simulink model "Virtual_Veh_Sim_EV3M_DLC"  (R2020a)
settings: configuration reference "Config_VarStep_Lat" (kept outside this file)
model workspace (MAT data in the model file):
  A = 159.22
  AccPwrbp = [0 0]
  AccSpdbp = [300 750]
  Aeff = 0.0314159265359
  Af = 2.46
  AfrStoich = 14.6
  AxlIxx = 62.3745166667
  AxlM = 160
  B = 1.01
  BattCapInit = 3.18
  BattCapInit_EV = 4.24
  BattChargeMax = 5.3
  BattChrgPwrMax = -60000
  BattChrgPwrMax_EV = -350000
  BattCurrMax = 300
  BattCurrMax_EV = 900
  BattDischrgPwrMax = 85000
  BattDischrgPwrMax_EV = 497000
  BattTempBp = [243.1 253.1 263.1 273.1 283.1 298.1 313.1]
  Battery : object (value not decoded)
  BrkPrsMax = 8273709
  Bx = 10
  C = 0.3618
  CapLUTBp = [0 0.01 0.02 0.03 0.04 0.05 0.06 0.07 0.08 0.09 0.1 0.11 ... (101 elements, 1x101)]
  CapSOCBp = [0 0.2 0.4 0.6 0.8 1]
  CatLightOffTime = 0
  Cd = 0.25
  ChrgLmt_bpt = [1 1 1 1 1 1 1 0.9 0.7 0.5 0]
  Cl = 0.1
  Cpm = 0.1
  Cps = 2
  CrankSpeed = 150
  Cx = 1.65
  Cz = 5565.2246438
  CzWhlAxl = 11490.971257
  DCT_Param : object (value not decoded)
  DischrgLmt_bpt = [0 0.5 0.7 0.9 1 1 1 1 1 1 1]
  Dn_Shft_Spd = [3 3 10 10 7 7 17 17 11 11 26 26 ... (20 elements, 4x5)]
  Downshift_Speeds = [9.5625 12.9375 16.3125 19.6875 23.0625 26.4375 29.8125 33.1875 36.5625 39.9375 43.3125 46.6875 ... (28 elements, 4x7)]
  Dx = 1
  ECMS_Ki = 0.1
  ECMS_Kp = 3
  ECMS_method = 1
  ECMS_s = 3.4
  Em = [2.8 3.228 3.284 3.361 3.408 3.427 3.472 3.477 3.493 3.504 3.516 3.528 ... (101 elements, 1x101)]
  EngStopStartEnable = 1
  EngStopTime : Simulink.Parameter (value not decoded)
  EngTrqCmd_0 = [0 5.91462851599 6.30130128159 6.63745773103 6.93103920513 7.1887141028 7.41614736865 7.6182009157 7.79908238179 7.96245469721 8.11151569725 8.24905488129 ... (21 elements, 1x21)]
  Ex = 0.01
  F0z = [2886 2907]
  F0zWhlAxl = 2907
  FZMAX = 6570
  FZMIN = 0
  Fc = 500
  FsbF = [-700000 -7000 -700 0 700 7000 700000]
  FsbR = [-700000 -7000 -700 0 700 7000 700000]
  FskF = [-8928.57142857 -178.571428571 0 357.142857143 535.714285714 9285.71428571]
  FskR = [-5357.14285714 -107.142857143 0 214.285714286 321.428571429 5571.42857143]
  G = [-1 0 1 2 3 4 5 6]
  G_o = 1
  Gear_Dn_bpt = [2 3 4 5 6]
  Gear_Up_bpt = [1 2 3 4 5]
  HEVEngTrq_min = 16.186104388
  Hmax = 0.25
  Iyy = 3000
  Iyy_Whl = 0.8
  J = 0.01
  J1 = 0.01
  J2 = 0.01
  Jd = 0.025
  Ji = 0.1
  Jin = 0.05
  Jin_Cltch = 0.2
  Jin_Cltch2 = 0.01
  Jout = [0.01 0.009 0.01 0.01 0.01 0.01 0.01 0.01]
  Jout_Cltch = 0.01
  Jout_Cltch2 = 0.05
  Jt = 0.1
  Jw1 = 0.01
  Jw2 = 0.01
  K_c = 10000
  Kpt = 12798
  Kz = 52451.0065793
  KzWhlAxl = 138031.612078
  LHV = 43000000
  Lhv = 42940000
  Lrel = 0.15
  Mass = 1623
  MaxTorque = [10.8721902117 76.2227873944 95.7133163788 115.203846226 134.694376076 154.184905918 173.675435766 181.839920951 181.509869828 181.17981871 180.849767971 180.519716854 ... (21 elements, 21x1)]
  N = [3.39 1 4.212 2.637 1.8 1.386 1 0.772]
  NCyl = 4
  NF = 2
  NR = 2
  N_P0 = 3
  N_P4 = 4.1
  N_idle = 750
  Ndiff = 3.32
  Ndiff_P4 = 4.1
  Ndiff_front = 5
  Ndiff_rear = 3.5
  Ndisk = 1
  Ndisks = 4
  Ngrid = 200
  Np = 2
  Np_EV = 35
  Np_FC = 1
  Ns = 72
  Ns_EV = 96
  Pabs = 101325
  Pdl_Pos_Dn_bpt = [0 0.6 0.9 1]
  Pdl_Pos_Up_bpt = [0 0.25 0.9 1]
  Pedal_Positions = [0.1 0.4 0.5 0.9]
  PenaltyFctr = 10000000
  Plimit = 60000
  Plimit_EV = 350000
  Press = 7000000
  Pstd = 101325
  RInt = [0.008846 0.006389 0.004364 0.002031 0.001443 0.0005603 0.001028 0.009319 0.006554 0.004101 0.002563 0.001825 ... (42 elements, 7x6)]
  Rair = 287
  Re = 0.327
  Reff = 0.11
  Reff_LSD = 0.2
  RegenBrkCutOff = [0 1]
  RegenBrkSpd_bpt = [2.2352 4.4704]
  Rm = 0.15
  SOCInit = 0.5
  SOCTrgt = 60
  SOC_bpt = [0 0.1 0.2 0.3 0.4 0.5 0.6 0.7 0.8 0.9 1]
  SOCmax = 80
  SOCmin = 40
  SUS : object (value not decoded)
  Sg = 0.743
  Sinj = 6.45161290323
  T = 273
  TCopy = 300
  T_eff_bp = [0 20 40 60 80 100 120 140 160 180 200]
  T_eff_bp_EV_front = [0 30 60 90 120 150 180 210 240 270 300]
  T_eff_bp_EV_rear = [0 20 40 60 80 100 120 140 160 180 200]
  T_eff_bp_P0 = [0 5.78745247607 6.36619772368 7.07355302631 7.95774715459 9.09456817668 10.6103295395 12.7323954474 15.9154943092 21.2206590789 66.6666666667]
  T_init = 298.15
  T_t = [200 200 200 200 190.9859317 143.2394488 114.591559 95.49296586 81.85111359 71.61972439 63.66197724 57.29577951 ... (14 elements, 1x14)]
  T_t_EV_front = [300 300 300 300 286.47889755 214.8591732 171.8873385 143.23944879 122.776670385 107.429586585 95.49296586 85.943669265 ... (14 elements, 1x14)]
  T_t_EV_rear = [200 200 200 200 190.9859317 143.2394488 114.591559 95.49296586 81.85111359 71.61972439 63.66197724 57.29577951 ... (14 elements, 1x14)]
  T_t_P0 = [66.6666666667 66.6666666667 66.6666666667 66.6666666667 21.2206590789 15.9154943092 12.7323954474 10.6103295395 9.09456817668 7.95774715459 7.07355302631 6.36619772368 ... (14 elements, 1x14)]
  Tc_Batt = 0.001
  Tc_DC = 0.001
  Tc_Mot = 0.02
  Temp_bpts = [313 358]
  TimeCnstECP = 0.125
  TimeCnstEGR = 0.125
  TimeCnstETC = 0.085
  TimeCnstICP = 0.125
  TimeCnstIVL = 0.125
  TimeCnstMFA = 0.125
  TimeCnstSWVA = 0.125
  TimeCnstVCR = 0.125
  TimeCnstVGT = 0.15
  TimeCnstVIRL = 0.125
  TimeCnstWGA = 0.15
  TimeStep = 0.0001
  TracPenaltyFctr = 50
  Trans : object (value not decoded)
  Trq_bpts = [25 50 75 100 150 200 250]
  Ts : Simulink.Parameter (value not decoded)
  Tstd = 293.15
  UNLOADED_RADIUS = 0.336
  Up_Shft_Spd = [5 5 12 12 9 9 19 19 13 13 28 28 ... (20 elements, 4x5)]
  Upshift_Speeds = [12.9375 16.3125 19.6875 33 26.4375 29.8125 33.1875 52.5 39.9375 43.3125 46.6875 77.25 ... (28 elements, 4x7)]
  VEH : object (value not decoded)
  VXLOW = 2
  Vd = 0.0015
  Vinit = 650
  WH : Mass (value not decoded)
  a = 3
  aMy = 0.01
  a_CG = 1.09
  afr_stoich = 14.6
  alphaMy = 0
  b : Simulink.Parameter (value not decoded)
  b1 = 100
  b1_g = 0.001
  b2 = 100
  b2_g = 0.001
  bMy = 0
  b_CG = 1.7
  b_J = 0.001
  bd = 0.001
  behavior = 0.2
  betaMy = 1
  bi = 0.001
  bin = 0.003
  bin_Cltch = 0.003
  bout = [0.003 0.003 0.003 0.003 0.003 0.003 0.003 0.003]
  bout_Cltch = 0.003
  br = 0.001
  bt = 0.001
  bw1 = 0.001
  bw2 = 0.001
  cMy = 0
  controller_type = 2
  defaultSpacing = 15
  disk_abore = 0.05
  domega_o = 0
  dt3D = 0.05
  dw = [0 10 20 40 60 80 100]
  dzdotsF = [-10 -1 -0.1 0 0.1 1 10]
  dzdotsR = [-10 -1 -0.1 0 0.1 1 10]
  dzsF = [-0.005 -0.0001 0 0.2 0.2001 0.2051]
  dzsR = [-0.005 -0.0001 0 0.2 0.2001 0.2051]
  eff = 98
  efficiency_table = [52 52 52 52 52 52 52 52 52 62 66 70 ... (154 elements, 14x11)]
  efficiency_table_EV = [85 85 85 85 85 85 85 85 85 85 85 85 ... (154 elements, 14x11)]
  efficiency_table_P0 = [52 52 52 52 52 52 52 52 52 62 66 70 ... (154 elements, 14x11)]
  egotf : object (value not decoded)
  elec_Pipe : object (value not decoded)
  elec_Radiator : object (value not decoded)
  eta = [0.95 0.95 0.95 0.95 0.95 0.95 0.95 0.95]
  eta_tbl = [0.7 0.8 0.9 0.9 0.9 0.9 0.9 0.7 0.8 0.9 0.9 0.9 ... (1232 elements, 7x11x8x2)]
  f_air = [0 0 0 0 0 0 0 0 0 0 0 0 ... (441 elements, 21x21)]
  f_co = [0 0 0 0 0 0 0 0 0 0 0 0 ... (441 elements, 21x21)]
  f_co2 = [0 0 0 0 0 0 0 0 0 0 0 0 ... (441 elements, 21x21)]
  f_cp_ld_bpt = [0 0.2 0.275 0.35 0.425 0.5 0.575 0.65 0.725 0.8 0.875 0.95 ... (16 elements, 1x16)]
  f_cp_n_bpt = [750 1053.57142857 1357.14285714 1660.71428571 1964.28571429 2267.85714286 2571.42857143 2875 3178.57142857 3482.14285714 3785.71428571 4089.28571429 ... (15 elements, 1x15)]
  f_del_sa_bpt = [0 0.75 1.5 2.25 3 3.75 4.5 5.25 6 6.75 7.5 8.25 ... (65 elements, 1x65)]
  f_ecp = [0 0 7.19012817097 15.3709456879 19.1470470057 19.0854874367 13.5819971805 0 0 0 0 0 ... (240 elements, 16x15)]
  f_eff = [499.877436556 432.508206156 399.540781628 370.894662993 347.954880181 331.11554878 319.468905906 311.408898718 305.523567029 300.961538912 297.204959405 293.79866205 ... (441 elements, 21x21)]
  f_egr_areapct_cmd = [0 3.448 6.897 10.34 13.79 17.24 20.69 24.14 27.59 31.03 34.48 37.93 ... (600 elements, 30x20)]
  f_egr_areapct_nrmlzdflow_bpt = [0 0.03448 0.06897 0.1034 0.1379 0.1724 0.2069 0.2414 0.2759 0.3103 0.3448 0.3793 ... (30 elements, 1x30)]
  f_egr_areapct_pr_bpt = [0.5 0.5263 0.5526 0.5789 0.6053 0.6316 0.6579 0.6842 0.7105 0.7368 0.7632 0.7895 ... (20 elements, 20x1)]
  f_egr_max_stdflow = [74.87 74.87 74.74 74.39 73.81 72.98 71.91 70.58 68.97 67.06 64.84 62.25 ... (20 elements, 1x20)]
  f_egr_stdflow = [0 3.743 7.487 11.23 14.97 18.72 22.46 26.2 29.95 33.69 37.43 41.18 ... (420 elements, 21x20)]
  f_egr_stdflow_egrap_bpt = [0 5 10 15 20 25 30 35 40 45 50 55 ... (21 elements, 21x1)]
  f_egr_stdflow_pr_bpt = [0.5 0.5263 0.5526 0.5789 0.6053 0.6316 0.6579 0.6842 0.7105 0.7368 0.7632 0.7895 ... (20 elements, 20x1)]
  f_egrpct_cmd = [0 0 0 0 0 0 0 0 0 0 0 0 ... (240 elements, 16x15)]
  f_egrpct_ld_bpt = [0 0.2 0.275 0.35 0.425 0.5 0.575 0.65 0.725 0.8 0.875 0.95 ... (16 elements, 1x16)]
  f_egrpct_n_bpt = [750 1054 1357 1661 1964 2268 2571 2875 3179 3482 3786 4089 ... (15 elements, 1x15)]
  f_fric_temp_bpt = [275 277 279 281 283 285 287 289 291 293 295 297 ... (46 elements, 1x46)]
  f_fric_temp_mod = [3.986 2.616 2.132 1.946 1.839 1.747 1.672 1.608 1.551 1.499 1.462 1.415 ... (46 elements, 1x46)]
  f_fuel = [0 0 0 0 0 0 0 0 0 0 0 0 ... (441 elements, 21x21)]
  f_hc = [0 0 0 0 0 0 0 0 0 0 0 0 ... (441 elements, 21x21)]
  f_icp = [0 0 1 1.09273642197 2.29409401139 3.54274371837 0.947749647567 0 0 0 0 0 ... (240 elements, 16x15)]
  f_intksys_stdflow_bpt = [0 29.67 59.34 89.01 117.8 144.1 155.7 166 175.2 183.3 190.7 197 ... (20 elements, 1x20)]
  f_intksys_stdflow_pr = [1 0.9789 0.9579 0.9368 0.9158 0.8947 0.8737 0.8526 0.8316 0.8105 0.7895 0.7684 ... (20 elements, 1x20)]
  f_lamcmd = [1 1 1 1 1 1 1 1 1 1 1 1 ... (240 elements, 16x15)]
  f_lamcmd_ld_bpt = [0 0.2 0.275 0.35 0.425 0.5 0.575 0.65 0.725 0.8 0.875 0.95 ... (16 elements, 1x16)]
  f_lamcmd_n_bpt = [750 1053.57142857 1357.14285714 1660.71428571 1964.28571429 2267.85714286 2571.42857143 2875 3178.57142857 3482.14285714 3785.71428571 4089.28571429 ... (15 elements, 1x15)]
  f_lcmd = [0 0.323404450126 0.402272754123 0.472190900601 0.545782048677 0.619112163094 0.619299299836 0.619299299836 0.619299299836 0.619299299836 0.619299299836 0.619299299836 ... (315 elements, 21x15)]
  f_lcmd_n_bpt = [750 1053.57142857 1357.14285714 1660.71428571 1964.28571429 2267.85714286 2571.42857143 2875 3178.57142857 3482.14285714 3785.71428571 4089.28571429 ... (15 elements, 1x15)]
  f_lcmd_tq_bpt = [0 15 25.2631578947 35.5263157895 45.7894736842 56.0526315789 66.3157894737 76.5789473684 86.8421052632 97.1052631579 107.368421053 117.631578947 ... (21 elements, 1x21)]
  f_m_lam = [0.94128 0.95565 0.97001 0.98437 0.99008 1.0004 0.97527 0.9549 0.92612 0.89735]
  f_m_lam_bpt = [0.65 0.7 0.75 0.8 0.85 0.9 0.95 1 1.05 1.1]
  f_m_sa = [1.0019 0.9988 0.9953 0.99173 0.98811 0.98441 0.98065 0.97682 0.97293 0.96897 0.96493 0.96083 ... (65 elements, 1x65)]
  f_mdot_air_corr = [1.02156051768 1.00597426471 0.989411677851 1.0033499089 0.984591437857 0.988509040623 1.0326198627 1.02765527362 1.0134784519 0.998280021213 0.981755128787 0.967218261288 ... (400 elements, 20x20)]
  f_mdot_air_corr_ld_bpt = [0.223381333333 0.285105122807 0.346828912281 0.408552701754 0.470276491228 0.532000280702 0.593724070175 0.655447859649 0.717171649123 0.778895438596 0.84061922807 0.902343017544 ... (20 elements, 1x20)]
  f_mdot_air_n_bpt = [750 973.6842 1197.3684 1421.0526 1644.7368 1868.4211 2092.1053 2315.7895 2539.4737 2763.1579 2986.8421 3210.5263 ... (20 elements, 1x20)]
  f_mdot_intk = [0 0 0 0 0 0 0 0 0 0 0 0 ... (400 elements, 20x20)]
  f_mdot_intk_ecp_bpt = [0 2.6316 5.2632 7.8947 10.5263 13.1579 15.7895 18.4211 21.0526 23.6842 26.3158 28.9474 ... (20 elements, 1x20)]
  f_mdot_trpd_bpt = [0 5.7895 11.5789 17.3684 23.1579 28.9474 34.7368 40.5263 46.3158 52.1053 57.8947 63.6842 ... (20 elements, 1x20)]
  f_nox = [0 0 0 0 0 0 0 0 0 0 0 0 ... (441 elements, 21x21)]
  f_nv = [0.64175366561 0.641419295169 0.640125365558 0.638690556197 0.644169906538 0.669178791311 0.731659452876 0.750078238889 0.750078238889 0.750078238889 0.750078238889 0.750078238889 ... (225 elements, 15x15)]
  f_nv_n_bpt = [750 1053.57142857 1357.14285714 1660.71428571 1964.28571429 2267.85714286 2571.42857143 2875 3178.57142857 3482.14285714 3785.71428571 4089.28571429 ... (15 elements, 1x15)]
  f_nv_prs_bpt = [31 40.6428571429 50.2857142857 59.9285714286 69.5714285714 79.2142857143 88.8571428571 98.5 108.142857143 117.785714286 127.428571429 137.071428571 ... (15 elements, 1x15)]
  f_pm = [0 0 0 0 0 0 0 0 0 0 0 0 ... (441 elements, 21x21)]
  f_sa = [9.05 9.05 16.4373253582 15.3405265461 13.6074880273 9.83352189562 3.89388784387 0 0 0 0 0 ... (240 elements, 16x15)]
  f_sa_ld_bpt = [0 0.2 0.275 0.35 0.425 0.5 0.575 0.65 0.725 0.8 0.875 0.95 ... (16 elements, 1x16)]
  f_sa_n_bpt = [750 1053.57142857 1357.14285714 1660.71428571 1964.28571429 2267.85714286 2571.42857143 2875 3178.57142857 3482.14285714 3785.71428571 4089.28571429 ... (15 elements, 1x15)]
  f_sa_opt = [35.3085 21.0105 10.3714 8.5076 7.1426 7.5656 -5.7766 -16.7061 -16.8345 -19.3546 -20.6085 -22.0872 ... (225 elements, 15x15)]
  f_startup_ect_bpt = [-40 0 20 50]
  f_startup_lambda_delta = [0.5 0.3 0.2 0]
  f_startup_lambda_delta_timecnst = [90 40 12 0]
  f_susp_axl_bp = [1 2]
  f_susp_dz_bp = [-0.325022776267 -0.315022776267 -0.305022776267 -0.205022776267 -0.105022776267 -0.00502277626717 0.0949772237328 0.194977223733 0.204977223733 0.214977223733]
  f_susp_dzdot_bp = [-3 -0.3 -0.2 -0.1 0 0.1 0.2 0.3 3]
  f_susp_fmz = [-144070.391448 -93629.24037 -75929.1118915 -20630.5828179 -15385.48216 -10140.3815021 -4895.28084414 349.819813785 -31916.3973792 18437.6709544 -83996.1993354 -33555.0482577 ... (43920 elements, 10x9x61x2x4)]
  f_susp_geom = [0 0 0 0 0 0 0 0 0 0 0 0 ... (3660 elements, 10x61x2x3)]
  f_susp_strgdelta_bp = [-0.523598775598 -0.506145483078 -0.488692190558 -0.471238898038 -0.453785605519 -0.436332312999 -0.418879020479 -0.401425727959 -0.383972435439 -0.366519142919 -0.349065850399 -0.331612557879 ... (61 elements, 1x61)]
  f_t_exh = [739.936218766 750.584766028 772.770773797 791.235245621 803.106549716 885.862998064 920.498479307 920.498479307 920.498479307 920.498479307 920.498479307 920.498479307 ... (225 elements, 15x15)]
  f_t_exh_l_bpt = [0.2 0.275 0.35 0.425 0.5 0.575 0.65 0.725 0.8 0.875 0.95 1.025 ... (15 elements, 1x15)]
  f_t_exh_n_bpt = [750 1053.57142857 1357.14285714 1660.71428571 1964.28571429 2267.85714286 2571.42857143 2875 3178.57142857 3482.14285714 3785.71428571 4089.28571429 ... (15 elements, 1x15)]
  f_tap = [0 0.9375 0.9375 0.982121188204 1.22093639741 1.5421156717 1.98870690459 2.59666257968 2.6875 2.6875 2.6875 2.6875 ... (315 elements, 21x15)]
  f_tap_ld_bpt = [0 0.2 0.268421052632 0.336842105263 0.405263157895 0.473684210526 0.542105263158 0.610526315789 0.678947368421 0.747368421053 0.815789473684 0.884210526316 ... (21 elements, 1x21)]
  f_tap_n_bpt = [750 1053.57142857 1357.14285714 1660.71428571 1964.28571429 2267.85714286 2571.42857143 2875 3178.57142857 3482.14285714 3785.71428571 4089.28571429 ... (15 elements, 1x15)]
  f_tbrake = [0 10.8721902117 10.8721902117 10.8721902117 10.8721902117 10.8721902117 10.8721902117 10.8721902117 10.8721902117 10.8721902117 10.8721902117 10.8721902117 ... (441 elements, 21x21)]
  f_tbrake_n_bpt = [0 750 973.684210526 1197.36842105 1421.05263158 1644.73684211 1868.42105263 2092.10526316 2315.78947368 2539.47368421 2763.15789474 2986.84210526 ... (21 elements, 1x21)]
  f_tbrake_t_bpt = [0 16.186104388 24.9146526824 33.6432009767 42.3717492711 51.1002975655 59.8288458599 68.5573941543 77.2859424487 86.0144907431 94.7430390375 103.471587332 ... (21 elements, 21x1)]
  f_texh = [630.359790352 638.212816583 644.85156876 656.410931683 676.180276582 706.880985433 749.880156186 804.757804763 869.00210738 938.264388175 1007.38061415 1071.70023123 ... (441 elements, 21x21)]
  f_tm_corr = [0.839360054391 0.833393271885 0.82629554201 0.818442814437 0.811524387436 0.809164184856 0.814606352881 0.826887956871 0.842304598924 0.856886829014 0.869487025783 0.880530414174 ... (400 elements, 20x20)]
  f_tm_corr_n_bpt = [750 973.6842 1197.3684 1421.0526 1644.7368 1868.4211 2092.1053 2315.7895 2539.4737 2763.1579 2986.8421 3210.5263 ... (20 elements, 1x20)]
  f_tm_corr_nd_bpt = [0.3 0.38947 0.47895 0.56842 0.65789 0.74737 0.83684 0.92632 1.0158 1.1053 1.1947 1.2842 ... (20 elements, 1x20)]
  f_tpp = [0 100]
  f_tpp_tap_bpt = [0 100]
  f_tq_fric = [4.16 4.42 4.69 4.88 4.94 4.93 4.85 4.74 4.63 4.52 4.42 4.34 ... (225 elements, 15x15)]
  f_tq_inr = [25.8508 37.8267 50.6081 62.6825 74.6026 88.9064 81.9508 76.6399 82.9886 85.0042 88.9209 92.7645 ... (225 elements, 15x15)]
  f_tq_inr_l_bpt = [0.2 0.28571 0.37143 0.45714 0.54286 0.62857 0.71429 0.8 0.88571 0.97143 1.0571 1.1429 ... (15 elements, 1x15)]
  f_tq_inr_n_bpt = [750 1053.5714 1357.1429 1660.7143 1964.2857 2267.8571 2571.4286 2875 3178.5714 3482.1429 3785.7143 4089.2857 ... (15 elements, 1x15)]
  f_tq_nl = [0 15.0012133443 26.4298333923 37.8556656512 49.2846782956 60.7113978793 72.3451969202 77.459652163 78.5324534074 78.5324534074 78.5324534074 78.5324534074 ... (256 elements, 16x16)]
  f_tq_nl_l_bpt = [0 0.2 0.275 0.35 0.425 0.5 0.575 0.65 0.725 0.8 0.875 0.95 ... (16 elements, 1x16)]
  f_tq_nl_n_bpt = [0 750 1053.57142857 1357.14285714 1660.71428571 1964.28571429 2267.85714286 2571.42857143 2875 3178.57142857 3482.14285714 3785.71428571 ... (16 elements, 1x16)]
  f_tq_pump = [7.24 5.67 3.94 2.59 1.8 1 1 1 1 1 1 1 ... (225 elements, 15x15)]
  f_twc_eff_co = [0.17 0.25 0.45 0.99 0.99 0.99 0.99]
  ... (+78 more variables)
symbols that are objects in the model workspace (value not decoded): VEH
undefined symbols (not defined in the file or in its folder): Disabled, DLCXref, DLCYref, Right, sigbuilder_block, SRE
libraries: simulink x11, vehdynlibscenariocommon x5, simulink_extras x5, vrlib x2, sim3dlib x2, vehdynlibviscommon x2, autolibshared x1, vehdynlibdriver x1, sim3dautolib x1
(part 4 of 6)

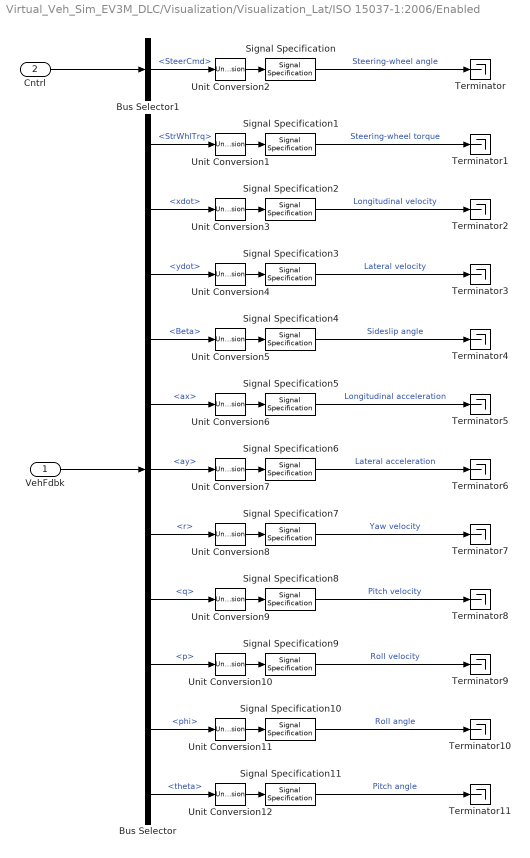
== system Virtual_Veh_Sim_EV3M_DLC/Visualization/Visualization_Lat/ISO 15037-1:2006/Enabled ==
  VehFdbk : Inport
  Cntrl : Inport  Port=2
  Bus Selector : BusSelector  OutputSignals=Steering.StrWhlTrq,Body.xdot,Body.ydot,Body.Beta,Body.ax,Body.ay,Body.r,Body.q,Body.p,Body.phi,Body.theta
  Bus Selector1 : BusSelector  OutputSignals=SteerCmd
  Signal Specification{,4,10..11} (4 alike) : SignalSpecification  Unit=deg
  Signal Specification1 : SignalSpecification  Unit=N*m
  Signal Specification2 : SignalSpecification  Unit=km/h
  Signal Specification3 : SignalSpecification  Unit=m/s
  Signal Specification5 : SignalSpecification  Unit=m/s^2
  Signal Specification6 : SignalSpecification  Unit=m/s^2
  Signal Specification7 : SignalSpecification  Unit=deg/s
  Signal Specification8 : SignalSpecification  Unit=deg/s
  Signal Specification9 : SignalSpecification  Unit=deg/s
  Terminator{,1..11} (12 alike) : Terminator
  Unit Conversion{1..12} (12 alike) : UnitConversion
  wires:
  Bus Selector/11 -> Unit Conversion12/1  "<theta>"
  Signal Specification11/1 -> Terminator11/1  "Pitch angle"
  Unit Conversion12/1 -> Signal Specification11/1
  Bus Selector/10 -> Unit Conversion11/1  "<phi>"
  Unit Conversion11/1 -> Signal Specification10/1
  Signal Specification10/1 -> Terminator10/1  "Roll angle"
  Bus Selector/9 -> Unit Conversion10/1  "<p>"
  Signal Specification9/1 -> Terminator9/1  "Roll velocity"
  Unit Conversion10/1 -> Signal Specification9/1
  Bus Selector/8 -> Unit Conversion9/1  "<q>"
  Unit Conversion9/1 -> Signal Specification8/1
  Signal Specification8/1 -> Terminator8/1  "Pitch velocity"
  Bus Selector/7 -> Unit Conversion8/1  "<r>"
  Signal Specification7/1 -> Terminator7/1  "Yaw velocity"
  Unit Conversion8/1 -> Signal Specification7/1
  Bus Selector/6 -> Unit Conversion7/1  "<ay>"
  Unit Conversion7/1 -> Signal Specification6/1
  Signal Specification6/1 -> Terminator6/1  "Lateral acceleration"
  Bus Selector/5 -> Unit Conversion6/1  "<ax>"
  Signal Specification5/1 -> Terminator5/1  "Longitudinal acceleration"
  Unit Conversion6/1 -> Signal Specification5/1
  Bus Selector/4 -> Unit Conversion5/1  "<Beta>"
  Unit Conversion5/1 -> Signal Specification4/1
  Signal Specification4/1 -> Terminator4/1  "Sideslip angle"
  Bus Selector/3 -> Unit Conversion4/1  "<ydot>"
  Signal Specification3/1 -> Terminator3/1  "Lateral velocity"
  Unit Conversion4/1 -> Signal Specification3/1
  Bus Selector/2 -> Unit Conversion3/1  "<xdot>"
  Unit Conversion3/1 -> Signal Specification2/1
  Signal Specification2/1 -> Terminator2/1  "Longitudinal velocity"
  Signal Specification1/1 -> Terminator1/1  "Steering-wheel torque"
  Unit Conversion1/1 -> Signal Specification1/1
  Bus Selector/1 -> Unit Conversion1/1  "<StrWhlTrq>"
  Signal Specification/1 -> Terminator/1  "Steering-wheel angle"
  Unit Conversion2/1 -> Signal Specification/1
  Bus Selector1/1 -> Unit Conversion2/1  "<SteerCmd>"
  Cntrl/1 -> Bus Selector1/1
  VehFdbk/1 -> Bus Selector/1

== system Virtual_Veh_Sim_EV3M_DLC/Visualization/Visualization_Lat/Scope Type/DLC ==
  VehFdbk : Inport
  Vis : Inport  Port=2
  Bus Creator : BusCreator  Inputs=3
  Bus Selector3 : BusSelector  OutputSignals=Veh.Body.Y,Veh.Body.X,Veh.Body.Z
  Bus Selector4 : BusSelector  OutputSignals=UB,LB,LtrlRef
  Lane Change : Scope  Commented=on
  Mux1 : Mux  Commented=on
  Signal Copy : SignalConversion  OverrideOpt=off
  Signal Copy1 : SignalConversion  OverrideOpt=off
  Signal Copy2 : SignalConversion  OverrideOpt=off
  Ref : Outport  VectorParamsAs1DForOutWhenUnconnected=off
  wires:
  Bus Selector4/1 -> Mux1/1  "<UB>"
  Bus Selector3/1 -> Mux1/4  "<Y>"
  VehFdbk/1 -> Bus Selector3/1
  Mux1/1 -> Lane Change/1
  Vis/1 -> Bus Selector4/1
  Bus Selector4/3 -> Signal Copy/1, Mux1/3  "<LtrlRef>"
  Bus Selector4/2 -> Mux1/2  "<LB>"
  Bus Selector3/2 -> Signal Copy1/1  "<X>"
  Bus Creator/1 -> Ref/1
  Bus Selector3/3 -> Signal Copy2/1  "<Z>"
  Signal Copy/1 -> Bus Creator/2  "YRef"
  Signal Copy1/1 -> Bus Creator/1  "XRef"
  Signal Copy2/1 -> Bus Creator/3  "ZRef"

== system Virtual_Veh_Sim_EV3M_DLC/Visualization/Visualization_Lat/Scope Type/None ==
  VehFdbk : Inport
  Vis : Inport  Port=2
  Cntrl : Inport  Port=3
  Bus Selector1 : BusSelector  OutputSignals=SteerCmd
  Bus Selector9 : BusSelector  OutputSignals=Veh.Body.r
  Signal Specification3 : SignalSpecification  Unit=deg/s
  Unit Conversion4 : UnitConversion
  Yaw Rate and Steer : Scope  NumInputPorts=2
  Ref : Outport  VectorParamsAs1DForOutWhenUnconnected=off
  wires:
  Bus Selector9/1 -> Unit Conversion4/1  "<r>"
  Signal Specification3/1 -> Yaw Rate and Steer/1
  Unit Conversion4/1 -> Signal Specification3/1
  VehFdbk/1 -> Bus Selector9/1  "VehFdbk"
  Bus Selector1/1 -> Yaw Rate and Steer/2  "<SteerCmd>"
  Vis/1 -> Ref/1
  Cntrl/1 -> Bus Selector1/1

== system Virtual_Veh_Sim_EV3M_DLC/Visualization/Visualization_Lat/Scope Type/XYZ ==
  VehFdbk : Inport
  Vis : Inport  Port=2
  Terminator : Terminator
  Ref : Outport  VectorParamsAs1DForOutWhenUnconnected=off
  wires:
  Vis/1 -> Ref/1
  VehFdbk/1 -> Terminator/1

== system Virtual_Veh_Sim_EV3M_DLC/Visualization/Visualization_Lat/Vehicle XY Plotter/XY View ==
  VehFdbk : Inport
  Bus Selector1 : BusSelector  OutputSignals=Veh.Body.phi,Veh.Body.theta,Veh.Body.psi  OutputAsBus=on
  Bus Selector5 : BusSelector  OutputSignals=Veh.Wheels.WhlAng  OutputAsBus=on
  Bus Selector6 : BusSelector  OutputSignals=Veh.Body.GeomX,Veh.Body.GeomY,Veh.Body.GeomZ  OutputAsBus=on
  Bus Selector7 : BusSelector  OutputSignals=Veh.Body.GeomXdot,Veh.Body.GeomYdot,Veh.Body.GeomZdot  OutputAsBus=on
  Bus to Vector : BusToVector
  Bus to Vector1 : BusToVector
  Bus to Vector2 : BusToVector
  Vehicle XY Plotter : Subsystem  mask(Vehicle XY Plotter){a=VEH.FrontAxlePositionfromCG, b=VEH.RearAxlePositionfromCG, w=VEH.TrackWidth, figBorder=10, bufferSize=1024, extRef=off, pltDT=.1}
      mask prompts: a "Distance to front axle from CG, a [m]:"; b "Distance to rear axle from CG, b [m]:"; w "Track width, w [m]:"; figBorder "Distance to figure borders, figBorder [m]:"; bufferSize "Path buffer sampe size, bufferSize []:"; extRef "Plot path reference, extRef"; pltDT "Plot update rate, pltDT [s]:"
      mask help:
      | This block will display a MATLAB figure which indicates the vehicle path, current position and heading velocity.
      | An optional path reference is also provided.
      mask init:
      | if autoblkschecksimstopped(gcb)
      |     PortName = 'RefXYZ';
      |     InportOption  = {'built-in/Ground', [PortName, ' Ground'];...
      |         'built-in/Inport',PortName };
      |     if ~strcmp(get_param(gcb,'extRef'),'on')
      |         NewBlkHdl = autoblksreplaceblock(gcb, InportOption, 1);
      |         set_param(NewBlkHdl, 'ShowName', 'off');
      |     else
      |         autoblksreplaceblock(gcb, InportOption, 2);
      |     end
      | end
      mask TypeOptions a: Vehicle XY Plotter/a
      mask TypeOptions b: Vehicle XY Plotter/b
      mask TypeOptions w: Vehicle XY Plotter/w
      mask TypeOptions figBorder: Vehicle XY Plotter/figBorder
      mask TypeOptions bufferSize: Vehicle XY Plotter/bufferSize
  wires:
  Bus to Vector2/1 -> Vehicle XY Plotter/2(InertAng)
  Bus to Vector/1 -> Vehicle XY Plotter/1(InertXYZ)
  Bus Selector5/1 -> Vehicle XY Plotter/4(delta)
  Bus Selector1/1 -> Bus to Vector2/1
  Bus Selector6/1 -> Bus to Vector/1
  Bus Selector7/1 -> Bus to Vector1/1
  VehFdbk/1 -> Bus Selector6/1, Bus Selector1/1, Bus Selector7/1, Bus Selector5/1
  Bus to Vector1/1 -> Vehicle XY Plotter/3(InertXdotYdotZdot)

== system Virtual_Veh_Sim_EV3M_DLC/Visualization/Visualization_Lat/Vehicle XY Plotter/XY View Ref ==
  VehFdbk : Inport
  Ref : Inport  Port=2
  Bus Selector1 : BusSelector  OutputSignals=Veh.Body.phi,Veh.Body.theta,Veh.Body.psi  OutputAsBus=on
  Bus Selector5 : BusSelector  OutputSignals=Veh.Wheels.WhlAng  OutputAsBus=on
  Bus Selector6 : BusSelector  OutputSignals=Veh.Body.GeomX,Veh.Body.GeomY,Veh.Body.GeomZ  OutputAsBus=on
  Bus Selector7 : BusSelector  OutputSignals=Veh.Body.GeomXdot,Veh.Body.GeomYdot,Veh.Body.GeomZdot  OutputAsBus=on
  Bus Selector8 : BusSelector  OutputSignals=XRef,YRef,ZRef  OutputAsBus=on
  Bus to Vector{,1..3} (4 alike) : BusToVector
  Vehicle XY Plotter : Subsystem  mask(Vehicle XY Plotter){a=VEH.FrontAxlePositionfromCG, b=VEH.RearAxlePositionfromCG, w=VEH.TrackWidth, figBorder=10, bufferSize=1024, extRef=on, pltDT=.1}
      mask prompts: a "Distance to front axle from CG, a [m]:"; b "Distance to rear axle from CG, b [m]:"; w "Track width, w [m]:"; figBorder "Distance to figure borders, figBorder [m]:"; bufferSize "Path buffer sampe size, bufferSize []:"; extRef "Plot path reference, extRef"; pltDT "Plot update rate, pltDT [s]:"
      mask help:
      | This block will display a MATLAB figure which indicates the vehicle path, current position and heading velocity.
      | An optional path reference is also provided.
      mask init: same as Virtual_Veh_Sim_EV3M_DLC/Visualization/Visualization_Lat/Vehicle XY Plotter/XY View/Vehicle XY Plotter
      mask TypeOptions a: Vehicle XY Plotter/a
      mask TypeOptions b: Vehicle XY Plotter/b
      mask TypeOptions w: Vehicle XY Plotter/w
      mask TypeOptions figBorder: Vehicle XY Plotter/figBorder
      mask TypeOptions bufferSize: Vehicle XY Plotter/bufferSize
  wires:
  Bus Selector8/1 -> Bus to Vector3/1
  Bus to Vector1/1 -> Vehicle XY Plotter/3(InertXdotYdotZdot)
  VehFdbk/1 -> Bus Selector5/1, Bus Selector7/1, Bus Selector1/1, Bus Selector6/1
  Bus Selector7/1 -> Bus to Vector1/1
  Bus Selector6/1 -> Bus to Vector/1
  Bus Selector1/1 -> Bus to Vector2/1
  Bus Selector5/1 -> Vehicle XY Plotter/4(delta)
  Bus to Vector/1 -> Vehicle XY Plotter/1(InertXYZ)
  Bus to Vector2/1 -> Vehicle XY Plotter/2(InertAng)
  Ref/1 -> Bus Selector8/1
  Bus to Vector3/1 -> Vehicle XY Plotter/5(RefXYZ)

== system Virtual_Veh_Sim_EV3M_DLC/Driver/Lateral Ref + DRV/Driver Commands/Driver Commands/Longitudinal Driver ==
  note: Balance = 0
      | Charge = 1
      | Driving = 2
  VehRef : Inport
  VehFdbk : Inport  Port=2
  Bus Creator1 : BusCreator  Inputs=9
  Bus Selector : BusSelector  OutputSignals=Veh.Body.xdot
  Bus Selector1 : BusSelector  OutputSignals=SteerOvrCmd,LngRef
  Constant5 : Constant  Value=false
  Constant6 : Constant  Value=0  OutDataTypeStr=double
  Constant7 : Constant  OutDataTypeStr=double
  Data Type Conversion : DataTypeConversion  OutDataTypeStr=boolean
  Dead Zone : DeadZone  LowerValue=-.1  UpperValue=.1  SaturateOnIntegerOverflow=on
  Enumerated Constant : simulink/Sources/Enumerated Constant  OutDataTypeStr=Enum: SRE  Value=SRE.Driving  SampleTime=inf
  Ground : Ground
  Ignition Switch Profile1 : Subsystem  Tag=STV Subsys  LoadFcn=sigbuilder_block('load');  StartFcn=sigbuilder_block('start');  StopFcn=sigbuilder_block('stop');  ClipboardFcn=sigbuilder_block('clipboard');  mask(Sigbuilder block){tuvar=[0:10]}
      mask help: Simulink:masks:SigbuilderBlock_MD
      mask init:
      | if ~strcmp(get_param(bdroot(gcbh),'SimulationStatus'),'stopped') tuvar = sigbuilder_block('maskInit'); end
      settings: CopyFcn=sigbuilder_block('copy');  DeleteFcn=sigbuilder_block('delete');  ModelCloseFcn=sigbuilder_block('modelClose');  PreSaveFcn=sigbuilder_block('preSave');  PauseFcn=sigbuilder_block('pause');  ContinueFcn=sigbuilder_block('continue');  NameChangeFcn=sigbuilder_block('namechange');  OpenFcn=sigbuilder_block('open',[595.8 176.4 550.8 322.2 ]);  CloseFcn=sigbuilder_block('close');
      mask Display: plot(0, 0, 100, 100,[2, 2, 32, 32, 2], [68, 8, 8, 68, 68],[32, 2], [38, 38], [32, 19, 2],[53, 60, 44], [32, 17, 17, 2],[16, 16, 31, 31]);txt = getActiveGroup(gcbh);text(2, 100, txt,'verticalAlignment', 'top');
  Longitudinal Driver : autolibshared/Longitudinal Driver  extAccelOvr=off  extDecelOvr=off  extAccelHld=off  extDecelHld=off  extAccelZero=off  extDecelZero=off  cntrlType=Predictive  shftType=None  velUnits=m/s  gearOut=on  Kp=5  Ki=5  Kff=.1  Kg=0  VehVelVec=[0 100]  KffVec=[.1 .1]  KpVec=[10 10]  KiVec=[5 5]  KgVec=[0 0]  m=VEH.Mass  Kpt=20000*1.5  tau=.5  L=3  aR=200  bR=2.5  cR=.5  g=9.81  vnom=5  Kaw=1  tauerr=.1  tauPt=2  GearInit=0  tShift=.1  pdlVec=[0.1 0.4 0.5 0.9]  upShftTbl=[-1 12.9375 26.4375 39.9375 51.18749999999999 62.4375 72.84375 83.25;-1 16.3125 29.8125 43.3125 54.5624 65.8125 76.78125 87.75;-1 19.6875 33.1875 46.68749999999999 57.9375 69.1875 80.71875 92.25;-1 33 52.5 77.25 100.5 138.75 161.875 185]  dwnShftTbl=[1 9.5625 23.0625 36.5625 47.8125 59.0625 68.90625 78.75;1 12.9375 26.4375 39.9375 51.18749999999999 62.4375 72.84375 83.25;1 16.3125 29.8125 43.3125 54.562499 65.8125 76.78125 87.75;1 19.6875 33.1875 46.68749999999999 57.9375 69.1875 80.71875 92.25]  tClutch=.5  tRev=.5  tPark=120  aMode=2  UpGearVec="[0  1  2  3  4  5  6  7]"  DownGearVec="[1  2  3  4  5  6  7  8]"
      settings: SourceProductBaseCode=PW,MT,VE,VP
  Manual Switch : ManualSwitch
  Manual Switch1 : ManualSwitch
  Optional Stationary Charging : Subsystem  Commented=on
  Signal Specification3 : SignalSpecification  Unit=rad
  Subsystem1 : Subsystem
  Terminator3 : Terminator
  Unit Conversion : UnitConversion
  Driver : Outport  VectorParamsAs1DForOutWhenUnconnected=off
  wires:
  Dead Zone/1 -> Longitudinal Driver/2
  Bus Creator1/1 -> Driver/1
  Unit Conversion/1 -> Signal Specification3/1
  Longitudinal Driver/3 -> Bus Creator1/3  "Decel"
  Longitudinal Driver/1 -> Terminator3/1
  Bus Selector1/2 -> Longitudinal Driver/1  "<LngRef>"
  VehRef/1 -> Bus Selector1/1
  VehFdbk/1 -> Bus Selector/1
  Bus Selector/1 -> Dead Zone/1  "<xdot>"
  Longitudinal Driver/2 -> Bus Creator1/2  "Accel"
  Ground/1 -> Longitudinal Driver/3
  Longitudinal Driver/4 -> Bus Creator1/4  "Gear"
  Bus Selector1/1 -> Unit Conversion/1  "<SteerOvrCmd>"
  Data Type Conversion/1 -> Manual Switch/2
  Constant7/1 -> Manual Switch1/2
  Ignition Switch Profile1/1(IGSW) -> Data Type Conversion/1
  Constant5/1 -> Manual Switch/1
  Optional Stationary Charging/1(Charge) -> Bus Creator1/7  "Chrg"
  Constant6/1 -> Manual Switch1/1
  Manual Switch/1 -> Bus Creator1/6  "IgSw"
  Manual Switch1/1 -> Bus Creator1/5  "AccEnbl"
  Signal Specification3/1 -> Bus Creator1/1  "SteerCmd"
  Subsystem1/1(ShiftCmd) -> Bus Creator1/8
  Enumerated Constant/1 -> Bus Creator1/9  "BMS_StateRequest"

== system Virtual_Veh_Sim_EV3M_DLC/Driver/Lateral Ref + DRV/Driver Commands/Driver Commands/Open Loop - F310 Gamepad ==
  note: Balance = 0
      | Charge = 1
      | Driving = 2
  VehFdbk : Inport
  Bus Creator1 : BusCreator  Inputs=10
  Enumerated Constant : simulink/Sources/Enumerated Constant  OutDataTypeStr=Enum: SRE  Value=SRE.Driving  SampleTime=inf
  Ground{,1..3} (4 alike) : Ground
  Joystick Input : vrlib/Joystick Input  joyid=1  adjustports=on  forcefeed=off
  Subsystem : Subsystem
  Subsystem1 : Subsystem
  Terminator : Terminator
  To Workspace1 : ToWorkspace  Commented=on  VariableName=str_ref  SaveFormat=Timeseries  SampleTime=.01
  To Workspace2 : ToWorkspace  Commented=on  VariableName=acc_ref  SaveFormat=Timeseries  SampleTime=.01
  To Workspace3 : ToWorkspace  Commented=on  VariableName=brk_ref  SaveFormat=Timeseries  SampleTime=.01
  Driver : Outport  VectorParamsAs1DForOutWhenUnconnected=off
  wires:
  VehFdbk/1 -> Subsystem1/1(VehFdbk)
  Subsystem1/3(Brake) -> To Workspace3/1, Bus Creator1/7  "Decel"
  Subsystem1/2(Accel) -> To Workspace2/1, Bus Creator1/6  "Accel"
  Subsystem1/4(Clutch) -> Bus Creator1/8
  Subsystem1/1(Steer) -> To Workspace1/1, Bus Creator1/5  "SteerCmd"
  Joystick Input/2 -> Subsystem/1(In1)
  Ground1/1 -> Bus Creator1/3  "xdotref"
  Ground2/1 -> Bus Creator1/2  "Chrg"
  Ground3/1 -> Bus Creator1/1  "IgSw"
  Ground/1 -> Bus Creator1/4  "AccEnbl"
  Subsystem/1(ShiftCmd) -> Bus Creator1/9  "ShiftCmd"
  Bus Creator1/1 -> Driver/1
  Joystick Input/1 -> Subsystem1/2(SteeringWheelAxes)  "SteeringWheelAxes"
  ? -> Terminator/1
  Enumerated Constant/1 -> Bus Creator1/10  "BMS_StateRequest"

== system Virtual_Veh_Sim_EV3M_DLC/Driver/Lateral Ref + DRV/Driver Commands/Driver Commands/Open Loop - G29 Steering Wheel and Pedals ==
  note: Balance = 0
      | Charge = 1
      | Driving = 2
  VehFdbk : Inport
  Bus Creator1 : BusCreator  Inputs=10
  Enumerated Constant : simulink/Sources/Enumerated Constant  OutDataTypeStr=Enum: SRE  Value=SRE.Driving  SampleTime=inf
  Ground{,1..3} (4 alike) : Ground
  Joystick Input : vrlib/Joystick Input  joyid=1  adjustports=on  forcefeed=off
  Subsystem1 : Subsystem
  Subsystem2 : Subsystem
  Terminator : Terminator
  To Workspace1 : ToWorkspace  Commented=on  VariableName=str_ref  SaveFormat=Timeseries  SampleTime=.01
  To Workspace2 : ToWorkspace  Commented=on  VariableName=acc_ref  SaveFormat=Timeseries  SampleTime=.01
  To Workspace3 : ToWorkspace  Commented=on  VariableName=brk_ref  SaveFormat=Timeseries  SampleTime=.01
  Driver : Outport  VectorParamsAs1DForOutWhenUnconnected=off
  wires:
  Joystick Input/1 -> Subsystem1/2(SteeringWheelAxes)  "SteeringWheelAxes"
  Bus Creator1/1 -> Driver/1
  Subsystem2/1(ShiftCmd) -> Bus Creator1/9  "ShiftCmd"
  Ground/1 -> Bus Creator1/4  "AccEnbl"
  Ground3/1 -> Bus Creator1/1  "IgSw"
  Ground2/1 -> Bus Creator1/2  "Chrg"
  Ground1/1 -> Bus Creator1/3  "xdotref"
  Joystick Input/2 -> Subsystem2/1(In1)
  Subsystem1/1(Steer) -> To Workspace1/1, Bus Creator1/5  "SteerCmd"
  Subsystem1/4(Clutch) -> Bus Creator1/8
  Subsystem1/2(Accel) -> To Workspace2/1, Bus Creator1/6  "Accel"
  Subsystem1/3(Brake) -> To Workspace3/1, Bus Creator1/7  "Decel"
  VehFdbk/1 -> Subsystem1/1(In1)
  ? -> Terminator/1
  Enumerated Constant/1 -> Bus Creator1/10  "BMS_StateRequest"

== system Virtual_Veh_Sim_EV3M_DLC/Driver/Lateral Ref + DRV/Driver Commands/Driver Commands/Open Loop Constant Radius ==
  VehFdbk : Inport
  SteerCmd : Inport  Port=2
  Accel : Inport  Port=3
  Brake : Inport  Port=4
  Gear : Inport  Port=5
  Bus Creator1 : BusCreator  Inputs=4
  Terminator : Terminator
  Unit Conversion{,1..3} (4 alike) : UnitConversion
  Wheel Angle Limit * Steer Ratio : Gain  Gain=40*pi/180*18
  Driver : Outport  VectorParamsAs1DForOutWhenUnconnected=off
  wires:
  Unit Conversion3/1 -> Bus Creator1/4  "Gear"
  Unit Conversion2/1 -> Bus Creator1/3  "Decel"
  Wheel Angle Limit * Steer Ratio/1 -> Bus Creator1/1  "SteerCmd"
  Bus Creator1/1 -> Driver/1
  Unit Conversion/1 -> Wheel Angle Limit * Steer Ratio/1
  Accel/1 -> Unit Conversion1/1
  VehFdbk/1 -> Terminator/1
  SteerCmd/1 -> Unit Conversion/1
  Unit Conversion1/1 -> Bus Creator1/2  "Accel"
  Brake/1 -> Unit Conversion2/1
  Gear/1 -> Unit Conversion3/1

== system Virtual_Veh_Sim_EV3M_DLC/Driver/Lateral Ref + DRV/Driver Commands/Driver Commands/Predictive Driver ==
  note: Balance = 0
      | Charge = 1
      | Driving = 2
  VehRef : Inport
  VehFdbk : Inport  Port=2
  Bus Creator1 : BusCreator  Inputs=9
  Bus Selector : BusSelector  OutputSignals=Veh.Body.xdot,Veh.Body.Y,Veh.Body.ydot,Veh.Body.psi,Veh.Body.r
  Bus Selector1 : BusSelector  OutputSignals=LngRef,LtrlRef,AccelZero
  Constant : Constant  Value=0
  Constant5 : Constant  Value=false
  Constant6 : Constant  Value=0  OutDataTypeStr=double
  Constant7 : Constant  OutDataTypeStr=double
  Data Type Conversion : DataTypeConversion  OutDataTypeStr=boolean
  Dead Zone : DeadZone  LowerValue=-.5  UpperValue=.5  ZeroCross=off  SaturateOnIntegerOverflow=on
  Dead Zone1 : DeadZone  LowerValue=-1e-2  UpperValue=1e-2  ZeroCross=off  SaturateOnIntegerOverflow=on
  Enumerated Constant : simulink/Sources/Enumerated Constant  Commented=on  OutDataTypeStr=Enum: SRE  Value=SRE.Driving  SampleTime=inf
  Ground : Ground
  Ignition Switch Profile1 : Subsystem  Tag=STV Subsys  LoadFcn=sigbuilder_block('load');  StartFcn=sigbuilder_block('start');  StopFcn=sigbuilder_block('stop');  ClipboardFcn=sigbuilder_block('clipboard');  mask(Sigbuilder block){tuvar=[0:10]}
      mask help: Simulink:masks:SigbuilderBlock_MD
      mask init:
      | if ~strcmp(get_param(bdroot(gcbh),'SimulationStatus'),'stopped') tuvar = sigbuilder_block('maskInit'); end
      settings: CopyFcn=sigbuilder_block('copy');  DeleteFcn=sigbuilder_block('delete');  ModelCloseFcn=sigbuilder_block('modelClose');  PreSaveFcn=sigbuilder_block('preSave');  PauseFcn=sigbuilder_block('pause');  ContinueFcn=sigbuilder_block('continue');  NameChangeFcn=sigbuilder_block('namechange');  OpenFcn=sigbuilder_block('open',[595.8 176.4 550.8 322.2 ]);  CloseFcn=sigbuilder_block('close');
      mask Display: plot(0, 0, 100, 100,[2, 2, 32, 32, 2], [68, 8, 8, 68, 68],[32, 2], [38, 38], [32, 19, 2],[53, 60, 44], [32, 17, 17, 2],[16, 16, 31, 31]);txt = getActiveGroup(gcbh);text(2, 100, txt,'verticalAlignment', 'top');
  Linear Predictive Driver : vehdynlibdriver/Predictive Driver  extAccelOvr=off  extDecelOvr=off  extAccelHld=off  extDecelHld=off  extAccelZero=off  extDecelZero=off  extSteerOvr=off  extSteerHld=off  extSteerZero=off  cntrlType=Predictive  shftType=Reverse, Neutral, Drive  velUnits=m/s  gearOut=on  steerOut=off  Kp=3  Ki=1  Kff=1  Kg=0  VehVelVec=[0 100]  KffVec=[.1 .1]  KpVec=[10 10]  KiVec=[5 5]  KgVec=[0 0]  vnom=5  Kaw=1  tauerr=.075  a=VEH.FrontAxlePositionfromCG  b=VEH.RearAxlePositionfromCG  m=VEH.Mass  I=VEH.YawMomentInertia  Cy_f=5000  Cy_r=7000  theta=30*pi/180  Ksteer=18  tau=0.03  L=6  Kpt=20000*5  aR=200  bR=2.5  cR=.5  g=9.81  GearInit=0  tShift=.1  pdlVec=[0.1 0.4 0.5 0.9]  upShftTbl=[-1 12.9375 26.4375 39.9375 51.18749999999999 62.4375 72.84375 83.25;-1 16.3125 29.8125 43.3125 54.5624 65.8125 76.78125 87.75;-1 19.6875 33.1875 46.68749999999999 57.9375 69.1875 80.71875 92.25;-1 33 52.5 77.25 100.5 138.75 161.875 185]  dwnShftTbl=[-1 12.9375 26.4375 39.9375 51.18749999999999 62.4375 72.84375 83.25;-1 16.3125 29.8125 43.3125 54.5624 65.8125 76.78125 87.75;-1 19.6875 33.1875 46.68749999999999 57.9375 69.1875 80.71875 92.25;-1 33 52.5 77.25 100.5 138.75 161.875 185]  tClutch=.5  tRev=.5  tPark=120  aMode=2  UpGearVec="[0  1  2  3  4  5  6  7]"  DownGearVec="[1  2  3  4  5  6  7  8]"
      settings: SourceProductBaseCode=VE
  Manual Switch : ManualSwitch
  Manual Switch1 : ManualSwitch
  Optional Stationary Charging : Subsystem  Commented=on
  Signal Specification3 : SignalSpecification  Unit=rad
  Subsystem1 : Subsystem
  Switch : Switch  Criteria=u2 > Threshold
  Terminator : Terminator
  Wheel Angle Limit * Steer Ratio : Gain  Gain=20*pi/180*18
  Driver : Outport  VectorParamsAs1DForOutWhenUnconnected=off
  wires:
  Switch/1 -> Bus Creator1/2  "Accel"
  Linear Predictive Driver/2 -> Dead Zone1/1
  Linear Predictive Driver/3 -> Switch/3
  Bus Selector/3 -> Linear Predictive Driver/6  "<ydot>"
  Ground/1 -> Linear Predictive Driver/3
  Constant/1 -> Switch/1
  Bus Selector/1 -> Dead Zone/1  "<xdot>"
  Bus Selector/2 -> Linear Predictive Driver/5  "<Y>"
  Bus Selector1/3 -> Switch/2  "<AccelZero>"
  Bus Creator1/1 -> Driver/1
  Dead Zone/1 -> Linear Predictive Driver/4
  Linear Predictive Driver/1 -> Terminator/1
  Bus Selector/4 -> Linear Predictive Driver/7  "<psi>"
  VehFdbk/1 -> Bus Selector/1
  Bus Selector1/2 -> Linear Predictive Driver/2  "<LtrlRef>"
  Bus Selector/5 -> Linear Predictive Driver/8  "<r>"
  Dead Zone1/1 -> Wheel Angle Limit * Steer Ratio/1
  VehRef/1 -> Bus Selector1/1
  Bus Selector1/1 -> Linear Predictive Driver/1  "<LngRef>"
  Wheel Angle Limit * Steer Ratio/1 -> Signal Specification3/1  "SteerCmd"
  Linear Predictive Driver/4 -> Bus Creator1/3  "Decel"
  Linear Predictive Driver/5 -> Bus Creator1/4  "Gear"
  Constant5/1 -> Manual Switch/1
  Ignition Switch Profile1/1(IGSW) -> Data Type Conversion/1
  Data Type Conversion/1 -> Manual Switch/2
  Manual Switch/1 -> Bus Creator1/6  "IgSw"
  Optional Stationary Charging/1(Charge) -> Bus Creator1/7  "Chrg"
  Constant6/1 -> Manual Switch1/1
  Manual Switch1/1 -> Bus Creator1/5  "AccEnbl"
  Constant7/1 -> Manual Switch1/2
  Signal Specification3/1 -> Bus Creator1/1
  Subsystem1/1(ShiftCmd) -> Bus Creator1/8
  Enumerated Constant/1 -> Bus Creator1/9  "BMS_StateRequest"

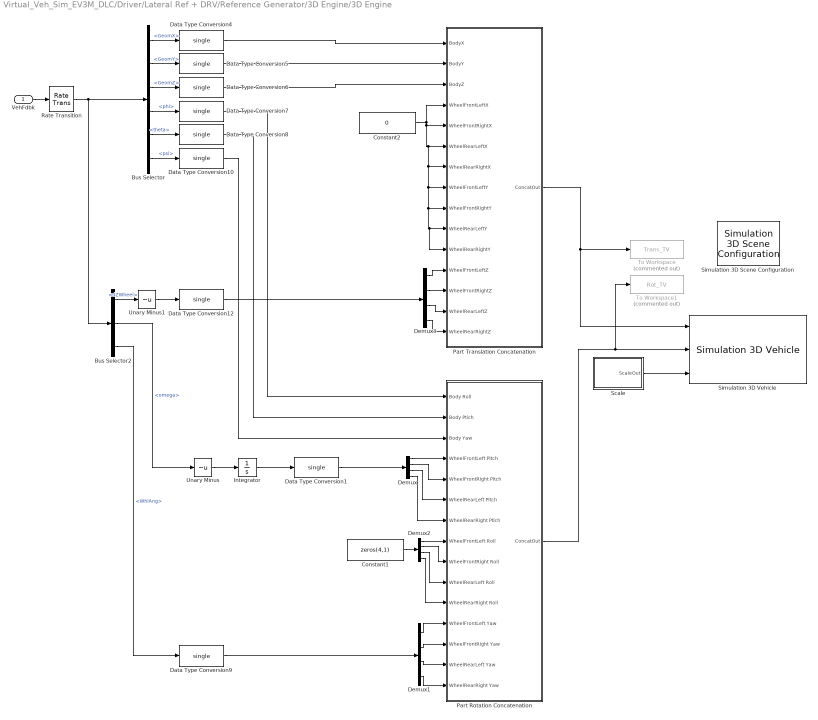
== system Virtual_Veh_Sim_EV3M_DLC/Driver/Lateral Ref + DRV/Reference Generator/3D Engine/3D Engine ==
  VehFdbk : Inport
  Bus Selector : BusSelector  OutputSignals=Veh.Body.GeomX,Veh.Body.GeomY,Veh.Body.GeomZ,Veh.Body.phi,Veh.Body.theta,Veh.Body.psi
  Bus Selector2 : BusSelector  OutputSignals=Veh.Wheels.dZWheel,Veh.Wheels.omega,Veh.Wheels.WhlAng
  Constant1 : Constant  Value=zeros(4,1)  OutDataTypeStr=single
  Constant2 : Constant  Value=0  OutDataTypeStr=single
  Data Type Conversion{1,4..10,12} (9 alike) : DataTypeConversion  OutDataTypeStr=single
  Demux{,1..3} (4 alike) : Demux
  Integrator : Integrator  WrapState=on  WrappedStateUpperValue=2*pi  WrappedStateLowerValue=0  ZeroCross=off
  Part Rotation Concatenation : Subsystem
  Part Translation Concatenation : Subsystem
  Rate Transition : RateTransition  OutPortSampleTime=dt3D
  Scale : Subsystem
  Simulation 3D Scene Configuration : sim3dlib/Simulation 3D Scene Configuration  Priority=0  ProjectFormat=Default Scenes  SceneDesc=Double lane change  ProjectName=VehicleSimulation.exe  ScenePath=/Game/Maps/HwStrght  vehTagList={'Scene Origin';'SimulinkVehicle1'}  vehTag=SimulinkVehicle1  OpVisEn=off  Ts=dt3D  EnableWindow=on  sensorTag=MainCamera4  sensorId=4  sensorName=MainCamera4  mountLoc=Origin  offsetFlag=off  tmountOffset=[0, 0, 0]  rmountOffset=[0, 0, 0]  HorizontalResolution=1280  VerticalResolution=720  HorizontalFOV=60  mountPoint=[0 0 0]  mountOrientation=[0 0 0]  aMode=aMode  ID=4
      settings: AttributesFormatString=Priority: %<Priority>  SourceProductBaseCode=DR,VE
  Simulation 3D Vehicle : sim3dautolib/Simulation 3D Vehicle  Priority=-1  PassVehMesh=Muscle car  VehColor=Red  ActorName=SimulinkVehicle1  Translation=[VEH.InitialLongPosition VEH.InitialLatPosition -VEH.InitialVertPosition; 0 0 0; 0 0 0; 0 0 0; 0 0 0]  Rotation=[VEH.InitialRollAngle VEH.InitialPitchAngle VEH.InitialYawAngle; 0 0 0; 0 0 0; 0 0 0; 0 0 0]  Scale=ones( 5, 3 )  SampleTime=dt3D  ActorType=SimulinkVehicle  ID=1  aMode=2  ActorTag=SimulinkVehicle1
      settings: SourceProductBaseCode=DR,VE
  To Workspace : ToWorkspace  Commented=on  VariableName=Trans_TV  SaveFormat=Timeseries  SampleTime=-1
  To Workspace1 : ToWorkspace  Commented=on  VariableName=Rot_TV  SaveFormat=Timeseries  SampleTime=-1
  Unary Minus : UnaryMinus
  Unary Minus1 : UnaryMinus
  wires:
  Unary Minus/1 -> Integrator/1
  Bus Selector2/1 -> Unary Minus1/1  "<dZWheel>"
  Rate Transition/1 -> Bus Selector/1, Bus Selector2/1
  Scale/1(ScaleOut) -> Simulation 3D Vehicle/3
  Demux/4 -> Part Rotation Concatenation/7(WheelRearRight Ptich)
  Demux/3 -> Part Rotation Concatenation/6(WheelRearLeft Pitch)
  Demux/2 -> Part Rotation Concatenation/5(WheelFrontRight Pitch)
  Demux/1 -> Part Rotation Concatenation/4(WheelFrontLeft Pitch)
  Constant1/1 -> Demux2/1
  Bus Selector/4 -> Data Type Conversion7/1  "<phi>"
  Data Type Conversion12/1 -> Demux3/1
  Demux3/4 -> Part Translation Concatenation/15(WheelRearRightZ)
  Demux3/3 -> Part Translation Concatenation/14(WheelRearLeftZ)
  Demux3/1 -> Part Translation Concatenation/12(WheelFrontLeftZ)
  Demux3/2 -> Part Translation Concatenation/13(WheelFrontRightZ)
  VehFdbk/1 -> Rate Transition/1
  Data Type Conversion6/1 -> Part Translation Concatenation/3(BodyZ)
  Demux1/4 -> Part Rotation Concatenation/15(WheelRearRight Yaw)
  Demux1/3 -> Part Rotation Concatenation/14(WheelRearLeft Yaw)
  Demux2/1 -> Part Rotation Concatenation/8(WheelFrontLeft Roll)
  Demux2/2 -> Part Rotation Concatenation/9(WheelFrontRight Roll)
  Demux2/3 -> Part Rotation Concatenation/10(WheelRearLeft Roll)
  Demux2/4 -> Part Rotation Concatenation/11(WheelRearRight Roll)
  Bus Selector2/3 -> Data Type Conversion9/1  "<WhlAng>"
  Bus Selector2/2 -> Unary Minus/1  "<omega>"
  Data Type Conversion9/1 -> Demux1/1
  Demux1/1 -> Part Rotation Concatenation/12(WheelFrontLeft Yaw)
  Demux1/2 -> Part Rotation Concatenation/13(WheelFrontRight Yaw)
  Integrator/1 -> Data Type Conversion1/1
  Data Type Conversion1/1 -> Demux/1
  Data Type Conversion8/1 -> Part Rotation Concatenation/2(Body Ptich)
  Data Type Conversion5/1 -> Part Translation Concatenation/2(BodyY)
  Data Type Conversion10/1 -> Part Rotation Concatenation/3(Body Yaw)
  Constant2/1 -> Part Translation Concatenation/5(WheelFrontRightX), Part Translation Concatenation/6(WheelRearLeftX), Part Translation Concatenation/7(WheelRearRightX), Part Translation Concatenation/8(WheelFrontLeftY), Part Translation Concatenation/9(WheelFrontRightY), Part Translation Concatenation/10(WheelRearLeftY), Part Translation Concatenation/11(WheelRearRightY), Part Translation Concatenation/4(WheelFrontLeftX)
  Data Type Conversion4/1 -> Part Translation Concatenation/1(BodyX)
  Data Type Conversion7/1 -> Part Rotation Concatenation/1(Body Roll)
  Bus Selector/1 -> Data Type Conversion4/1  "<GeomX>"
  Bus Selector/2 -> Data Type Conversion5/1  "<GeomY>"
  Bus Selector/6 -> Data Type Conversion10/1  "<psi>"
  Bus Selector/5 -> Data Type Conversion8/1  "<theta>"
  Bus Selector/3 -> Data Type Conversion6/1  "<GeomZ>"
  Unary Minus1/1 -> Data Type Conversion12/1
  Part Rotation Concatenation/1(ConcatOut) -> To Workspace1/1, Simulation 3D Vehicle/2
  Part Translation Concatenation/1(ConcatOut) -> Simulation 3D Vehicle/1, To Workspace/1

== system Virtual_Veh_Sim_EV3M_DLC/Driver/Lateral Ref + DRV/Reference Generator/3D Engine/3D Engine Disabled ==
  VehFdbk : Inport
  Terminator : Terminator
  wires:
  VehFdbk/1 -> Terminator/1

== system Virtual_Veh_Sim_EV3M_DLC/Driver/Lateral Ref + DRV/Reference Generator/Reference Generator/Double Lane Change ==
  "VehFdbk " : Inport
  Double Lane Change : vehdynlibscenariocommon/Lane Change Reference Generator  VariantControl=Variant1  t_start=t_start  XGate=XGate  xdot_r=xdot_r  xdotUnit=mph  xStart=xStart  vehW=vehW  lattoff=lattoff  centerSwitch=on  latRefbp=latRefbp  latRef=latRef  aMode=2
      settings: SourceProductBaseCode=VE
  " Vis" : Outport  VectorParamsAs1DForOutWhenUnconnected=off
  " Ref" : Outport  Port=2  VectorParamsAs1DForOutWhenUnconnected=off
  " Fdbk" : Outport  Port=3  VectorParamsAs1DForOutWhenUnconnected=off
  wires:
  Double Lane Change/2 -> " Ref"/1
  Double Lane Change/1 -> " Vis"/1
  "VehFdbk "/1 -> Double Lane Change/1, " Fdbk"/1

== system Virtual_Veh_Sim_EV3M_DLC/Driver/Lateral Ref + DRV/Reference Generator/Reference Generator/Increasing Steer ==
  "VehFdbk " : Inport
  Bus Creator : BusCreator  Inputs=3
  Ground : Ground
  Ground1 : Ground
  Ground2 : Ground
  Increasing Steer : vehdynlibscenariocommon/Slowly Increasing Steer  VariantControl=1  t_start=t_start  xdot_r=xdot_r  xdotUnit=mph  omega_hw=omega_hw  theta_max=theta_max  t_stop=t_stop  ay_max=ay_max  ay_stop=off  aMode=2
      settings: SourceProductBaseCode=VE
  " Vis" : Outport  VectorParamsAs1DForOutWhenUnconnected=off
  " Ref" : Outport  Port=2  VectorParamsAs1DForOutWhenUnconnected=off
  " Fdbk" : Outport  Port=3  VectorParamsAs1DForOutWhenUnconnected=off
  wires:
  Ground/1 -> Bus Creator/1  "XRef"
  Ground1/1 -> Bus Creator/2  "YRef"
  Ground2/1 -> Bus Creator/3  "ZRef"
  Increasing Steer/1 -> " Ref"/1  "LtrlRef"
  Bus Creator/1 -> " Vis"/1
  "VehFdbk "/1 -> Increasing Steer/1, " Fdbk"/1

== system Virtual_Veh_Sim_EV3M_DLC/Driver/Lateral Ref + DRV/Reference Generator/Reference Generator/Open Loop - F310 Gamepad ==
  "VehFdbk " : Inport
  Bus Creator : BusCreator  Inputs=3
  Ground{,1..3} (4 alike) : Ground
  " Vis" : Outport  VectorParamsAs1DForOutWhenUnconnected=off
  " Ref" : Outport  Port=2  VectorParamsAs1DForOutWhenUnconnected=off
  " Fdbk" : Outport  Port=3  VectorParamsAs1DForOutWhenUnconnected=off
  wires:
  Ground3/1 -> " Ref"/1
  Ground/1 -> Bus Creator/1  "XRef"
  Ground1/1 -> Bus Creator/2  "YRef"
  Ground2/1 -> Bus Creator/3  "ZRef"
  Bus Creator/1 -> " Vis"/1
  "VehFdbk "/1 -> " Fdbk"/1
